simulink model "lab"  (R2018b)
settings: Solver=VariableStepAuto  StartTime=0.0  StopTime=100  RelTol=1e-3
InitFcn:
  | [num,den] = tfdata(C);
  | num=cell2mat(num);
  | kd=num(1,1);
  | kp=num(1,2);
  | ki=num(1,3);
  | s=.0177; % area
  | h=.108; % height
  | v0=.0075;%area*height
  | k=140*2*(sqrt(s*v0))
settings Model: Creator=exx241  LastModifiedBy=Matteo Cecamore

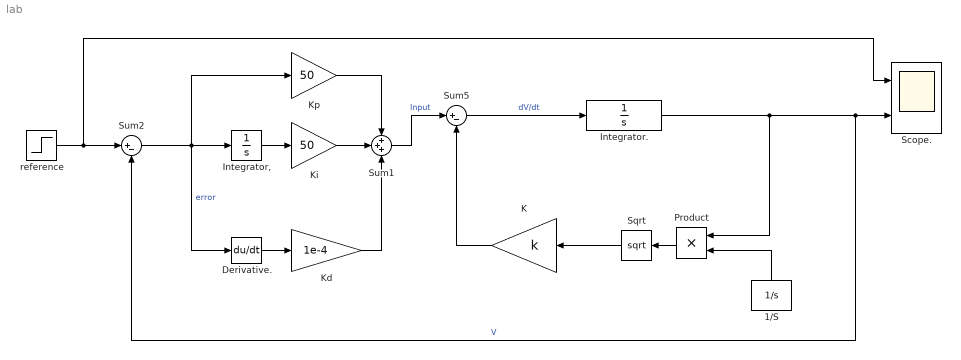
== system lab ==
  1/S : Constant  Value=1/s
  Derivative. : Derivative
  Integrator, : Integrator
  Integrator. : Integrator
  K : Gain  Gain=k
  Kd : Gain  Gain=1e-4
  Ki : Gain  Gain=50
  Kp : Gain  Gain=50
  Product : Product
  Scope. : Scope  NumInputPorts=2
  Sqrt : Sqrt  SaturateOnIntegerOverflow=on
  Sum1 : Sum  Inputs=+++
  Sum2 : Sum  Inputs=|+-
  Sum5 : Sum  Inputs=|+-
  reference : Step  After=.001  SampleTime=0
  wires:
  Sum5/1 -> Integrator./1  "dV/dt"
  1/S/1 -> Product/2
  Product/1 -> Sqrt/1
  Sqrt/1 -> K/1
  K/1 -> Sum5/2
  Integrator./1 -> Sum2/2, Scope./2, Product/1  "V"
  Kp/1 -> Sum1/1
  Ki/1 -> Sum1/2
  Kd/1 -> Sum1/3
  Sum2/1 -> Kp/1, Integrator,/1, Derivative./1  "error"
  Derivative./1 -> Kd/1
  Integrator,/1 -> Ki/1
  reference/1 -> Scope./1, Sum2/1
  Sum1/1 -> Sum5/1  "Input"
